simulink model "ADAS_Brake_Con_TS8"  (Simulink 5.0)
settings: Solver=ode45  SolverMode=SingleTasking  StartTime=0  StopTime=8  FixedStep=0.002  RelTol=1e-3  AbsTol=1e-6
libraries: Solver_SF x1
settings Model: Creator=pmather  LastModifiedBy=ywata  ExtModeTrigMode=oneshot  ExtModeArmWhenConnect=off  LimitDataPoints=off  BlockReductionOpt=off  BooleanDataType=off  RTWTemplateMakefile=grt_vc.tmf  RTWOptions="-aEnforceIntegerDowncast=1 -aFoldNonRolledExpr=1 -aInlineInvariantSignals=0 -aInlineParameters=0 -aLocalBlockOutputs=1 -aRollThreshold=5 -aZeroInternalMemoryAtStartup=1 -aZeroExternalMemoryAtStartup=1 -aInitFltsAndDblsToZero=1 -aGenerateReport=0 -aGenCodeOnly=0 -aRTWVerbose=1 -aIncludeHyperlinkInReport=0 -aLaunchReport=0 -aForceParamTrailComments=0 -aGenerateComments=1 -aIgnoreCustomStorageClasses=1 -aIncHierarchyInIds=0 -aMaxRTWIdLen=31 -aShowEliminatedStatements=0 -aPrefixModelToSubsysFcnNames=1 -aIncDataTypeInIds=0 -aInsertBlockDesc=0 -aSimulinkBlockComments=1 -aInlinedPrmAccess=\"Literals\"  -aSuppressErrorStatus=0 -aModelReferenceCompliant=1 -aParenthesesLevel=\"Nominal\" -aModelStepFunctionPrototypeControlCompliant=0 -aPortableWordSizes=0 -aSupportNonInlinedSFcns=1 -aSupportContinuousTime=1 -aSupportComplex=1 -aSupportNonFinite=1 -aSupportAbsoluteTime=1 -aTargetPreCompLibLocation=\"\" -aTargetLibSuffix=\"\" -aTargetFcnLib=\"ansi_tfl_tmw.mat\" -aMultiInstanceERTCode=0 -aLogVarNameModifier=\"rt_\" -aIsPILTarget=0 -aCombineOutputUpdateFcns=0 -aGenerateASAP2=0 -aGenerateClassInterface=0 -aGenerateTestInterfaces=0 -aGenerateSampleERTMain=0 -aGenerateFullHeader=1 -aUtilityFuncGeneration=\"Auto\" -aIncludeFileDelimiter=\"Auto\" -aIncludeMdlTerminateFcn=1 -aPurelyIntegerCode=0 -aERTCustomFileBanners=0 -aRTWCAPIStates=0 -aRTWCAPIParams=0 -aRTWCAPISignals=0 -aMatFileLogging=1 -aGenFloatMathFcnCalls=\"ANSI_C\" -aExtModeMexFile=\"ext_comm\" -aExtModeTransport=0 -aExtModeStaticAllocSize=1000000 -aExtModeTesting=0 -aExtModeStaticAlloc=0 -aExtMode=0"

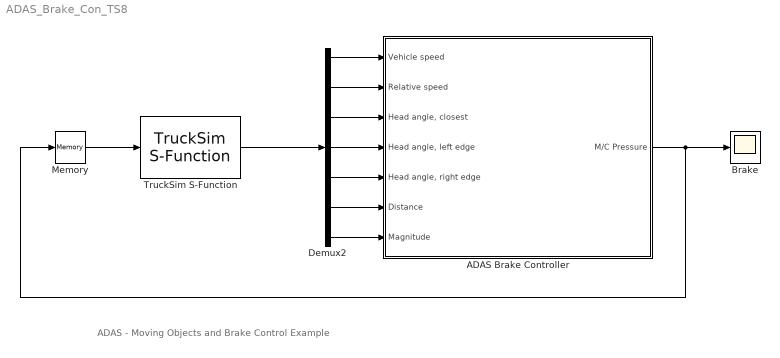
== system ADAS_Brake_Con_TS8 ==
  note: ADAS - Moving Objects and Brake Control Example
  ADAS Brake Controller : Subsystem
  Brake : Scope
      settings: TimeRange=8  YMin=0  YMax=15  SaveName=ScopeData2
  Demux2 : Demux  Outputs=7
  Memory : Memory
  TruckSim S-Function : Solver_SF/TruckSim S-Function  Priority=1  AncestorBlock=Solver_SF/CarSim S-Function  VehicleCode=???
      settings: AttributesFormatString=Vehicle Code: %<VehicleCode>
  wires:
  Memory/1 -> TruckSim S-Function/1
  ADAS Brake Controller/1(M/C Pressure) -> Memory/1, Brake/1
  TruckSim S-Function/1 -> Demux2/1
  Demux2/1 -> ADAS Brake Controller/1(Vehicle speed)
  Demux2/2 -> ADAS Brake Controller/2(Relative speed)
  Demux2/3 -> ADAS Brake Controller/3("Head angle, closest")
  Demux2/4 -> ADAS Brake Controller/4("Head angle, left edge ")
  Demux2/5 -> ADAS Brake Controller/5("Head angle, right edge")
  Demux2/6 -> ADAS Brake Controller/6(Distance)
  Demux2/7 -> ADAS Brake Controller/7(Magnitude)

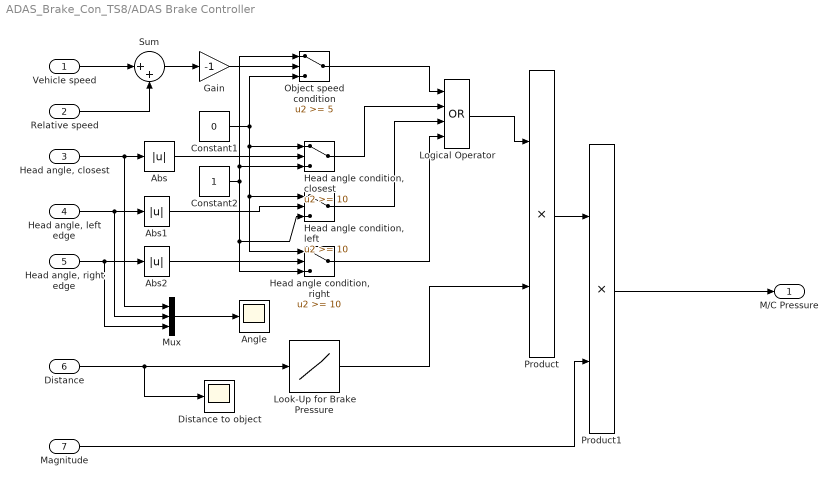
== system ADAS_Brake_Con_TS8/ADAS Brake Controller ==
  Vehicle speed : Inport
  Relative speed : Inport  Port=2
  "Head angle, closest" : Inport  Port=3
  "Head angle, left edge " : Inport  Port=4
  "Head angle, right edge" : Inport  Port=5
  Distance : Inport  Port=6
  Magnitude : Inport  Port=7
  Abs : Abs  SaturateOnIntegerOverflow=on
  Abs1 : Abs  SaturateOnIntegerOverflow=on
  Abs2 : Abs  SaturateOnIntegerOverflow=on
  Angle : Scope
      settings: TimeRange=8  YMin=0  YMax=100  SaveName=ScopeData3
  Constant1 : Constant  Value=0
  Constant2 : Constant
  Distance to object : Scope
      settings: TimeRange=8  YMin=0  YMax=150  SaveName=ScopeData4
  Gain : Gain  Gain=-1  SaturateOnIntegerOverflow=on
  "Head angle condition, closest" : Switch  Threshold=10  SaturateOnIntegerOverflow=on  InputSameDT=on
  "Head angle condition, left" : Switch  Threshold=10  SaturateOnIntegerOverflow=on  InputSameDT=on
  "Head angle condition, right" : Switch  Threshold=10  SaturateOnIntegerOverflow=on  InputSameDT=on
  Logical Operator : Logic  Operator=OR  Inputs=4
  Look-Up for Brake Pressure : Lookup  InputValues=[0,20,30,40,60,80,100,120]  OutputValues=[15,15,10,10,0,0,0,0]  SaturateOnIntegerOverflow=on
  Mux : Mux  Inputs=3
  Object speed condition : Switch  Threshold=5  SaturateOnIntegerOverflow=on  InputSameDT=on
  Product : Product  SaturateOnIntegerOverflow=on  InputSameDT=on
  Product1 : Product  SaturateOnIntegerOverflow=on  InputSameDT=on
  Sum : Sum  Inputs=|++  SaturateOnIntegerOverflow=on  InputSameDT=on
  M/C Pressure : Outport
  wires:
  Abs/1 -> "Head angle condition, closest"/2
  Constant1/1 -> Object speed condition/3, "Head angle condition, closest"/1, "Head angle condition, left"/1, "Head angle condition, right"/1
  Constant2/1 -> "Head angle condition, closest"/3, Object speed condition/1, "Head angle condition, left"/3, "Head angle condition, right"/3
  Sum/1 -> Gain/1
  Gain/1 -> Object speed condition/2
  Object speed condition/1 -> Logical Operator/1
  "Head angle condition, closest"/1 -> Logical Operator/2
  Logical Operator/1 -> Product/1
  Look-Up for Brake Pressure/1 -> Product/2
  Product/1 -> Product1/1
  Vehicle speed/1 -> Sum/1
  Relative speed/1 -> Sum/2
  "Head angle, closest"/1 -> Abs/1, Mux/1
  Distance/1 -> Look-Up for Brake Pressure/1, Distance to object/1
  Product1/1 -> M/C Pressure/1
  "Head angle, left edge "/1 -> Abs1/1, Mux/2
  "Head angle, right edge"/1 -> Abs2/1, Mux/3
  "Head angle condition, left"/1 -> Logical Operator/3
  Magnitude/1 -> Product1/2
  Mux/1 -> Angle/1
  Abs1/1 -> "Head angle condition, left"/2
  Abs2/1 -> "Head angle condition, right"/2
  "Head angle condition, right"/1 -> Logical Operator/4
